simulink model "Voltage_calculation"  (R2022b)
settings: Solver=ode4  StartTime=1  StopTime=5000  FixedStep=1  MaxStep=250  RelTol=1e-3
model workspace (MAT data in the model file):
  Voltage_calculation_spesession : sldodialogs.data.SessionData (value not decoded)
values from neighbouring files (symbols this model uses):
  sigma_neg = 0.17    [sigma_neg.mat]
  sigma_pos = 100    [sigma_pos.mat]
settings Model: Creator=sus-ap  LastModifiedBy=sus-ap
settings DataIOCC: ExternalInput=[T i_app V_app phis_pos phis_neg]  LoadExternalInput=on  SaveFormat=Array  SignalLogging=off  DSMLogging=off  ReturnWorkspaceOutputs=off  OutputTimes=SDO_OutputTimes  ReturnWorkspaceOutputsName=SDOSimTest_Log  DatasetSignalFormat=timetable  LoggingIntervals=[0, 250]
settings ModelReferenceCC: PropagateSignalLabelsOutOfModel=off

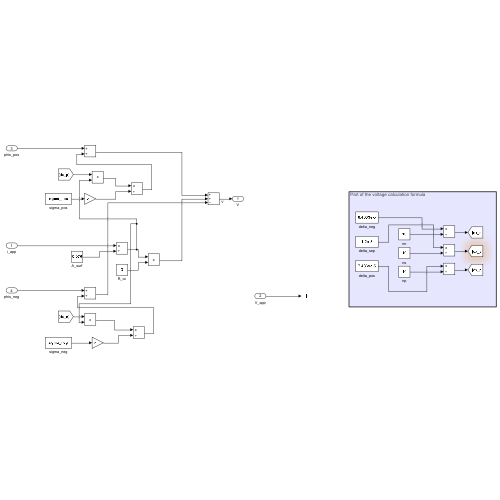
[thumbnail: Simulink's stored preview of the top-level diagram]
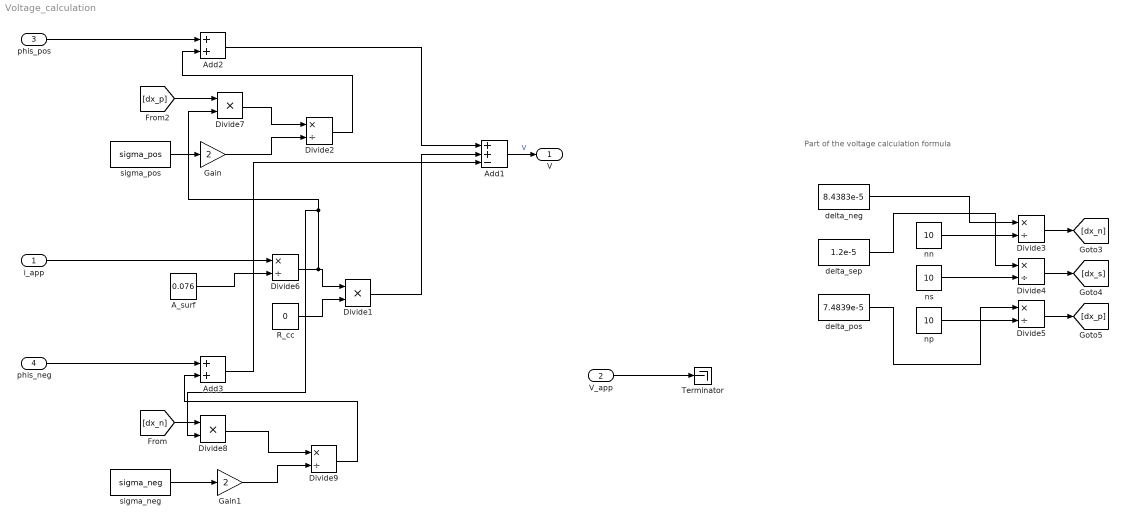
== system Voltage_calculation ==
  note: Part of the voltage calculation formula
  i_app : Inport
  V_app : Inport  Port=2
  phis_pos : Inport  Port=3
  phis_neg : Inport  Port=4
  A_surf : Constant  Value=0.076
  Add1 : Sum  Inputs=++-
  Add2 : Sum
  Add3 : Sum
  Divide1 : Product  Inputs=**
  Divide{2..6,9} (6 alike) : Product  Inputs=*/
  Divide7 : Product  Inputs=**
  Divide8 : Product  Inputs=**
  Gain : Gain  Gain=2
  Gain1 : Gain  Gain=2
  R_cc : Constant  Value=0
  Terminator : Terminator
  delta_neg : Constant  Value=8.4383e-5
  delta_pos : Constant  Value=7.4839e-5
  delta_sep : Constant  Value=1.2e-5
  nn : Constant  Value=10
  np : Constant  Value=10
  ns : Constant  Value=10
  sigma_neg : Constant  Value=sigma_neg
  sigma_pos : Constant  Value=sigma_pos
  V : Outport
  wires:
  V_app/1 -> Terminator/1
  Gain1/1 -> Divide9/2
  delta_pos/1 -> Divide5/1
  delta_neg/1 -> Divide3/1
  nn/1 -> Divide3/2
  Divide3/1 -> [dx_n]
  [dx_p] -> Divide7/1
  Divide7/1 -> Divide2/1
  delta_sep/1 -> Divide4/1
  i_app/1 -> Divide6/1
  np/1 -> Divide5/2
  sigma_neg/1 -> Gain1/1
  phis_neg/1 -> Add3/1
  ns/1 -> Divide4/2
  A_surf/1 -> Divide6/2
  Gain/1 -> Divide2/2
  [dx_n] -> Divide8/1
  sigma_pos/1 -> Gain/1
  R_cc/1 -> Divide1/2
  Add3/1 -> Add1/3
  Divide1/1 -> Add1/2
  Divide5/1 -> [dx_p]
  Divide4/1 -> [dx_s]
  Divide2/1 -> Add2/2
  Divide9/1 -> Add3/2
  Add2/1 -> Add1/1
  Divide6/1 -> Divide8/2, Divide7/2, Divide1/1
  Divide8/1 -> Divide9/1
  phis_pos/1 -> Add2/1
  Add1/1 -> V/1  "V"
